simulink model "SDV_HIL"  (R2025a)
settings: Solver=VariableStepAuto  StartTime=0.0  StopTime=9999  FixedStep=0.001  RelTol=1e-3
undefined symbols (not defined in the file): Breakpoints_Fz, Cij, dspblkCoreblockFVToolHelper, eta, Fx_total_max, g, gcbh, Iz, lambda, lf, lr, mu, phi, R_eff, Tmax, xi
libraries: simulink_extras x30, slrealtimeiplib x17, slpidlib x16, simulink x10, SignalEditorBlockLib x6, dspstat3 x5, Solver_SF x3, sl3dlib x3
(part 5 of 5)

== matlab function SDV_HIL/Draft1/Steering Input1/Driver Logi G29/MATLAB Function ==
  data: btn input; state output
function state = fnc(btn)
%#codegen
% Start/Stop toggle dari 1 tombol joystick
% btn  : input tombol (0 atau 1, tipe double)
% state: output status (0=stop, 1=start)

persistent s last
if isempty(s)
    s = 0;      % status awal stop
    last = 0;   % tombol sebelumnya
end

% pastikan semua double
btn  = double(btn);
s    = double(s);
last = double(last);

% deteksi rising edge
if (btn == 1) && (last == 0)
    s = 1 - s;  % toggle
end

% simpan status tombol sebelumnya
last = btn;

% keluaran status
state = s;
end

== matlab function SDV_HIL/Draft1/UDP Receive ZCU -> PC1/MATLAB Function ==
  data: payload input; FL output; FR output; RL output; RR output; seqRecv output
function [FL, FR, RL, RR, seqRecv] = recvZCUFrame(payload)

% -------------------------------------------------------------------------
% recvZCUFrame
% Receive UDP frame from ZCU and decode per-wheel data
%
% Frame format (7 bytes):
% [1] Header = 0xCA
% [2] ID     = 1..4
% [3:4] Speed (int16)
% [5:6] Angle (int16)
% [7] Seq    (uint8)
% -------------------------------------------------------------------------

% =======================
% Persistent storage

persistent data
if isempty(data)
    % data(row,:) = [angle speed seq]
    data = zeros(4,3,'double');
end

% =======================
% Process incoming payload

data = processOne(payload, data);

% =======================
% Outputs

FL = data(1,1:2);
FR = data(2,1:2);
RL = data(3,1:2);
RR = data(4,1:2);

seqRecv = data(:,3);

% =======================
% Nested function

    function dataOut = processOne(payloadIn, dataIn)

        dataOut = dataIn;

        % Length check
        if numel(payloadIn) < 7
            return;
        end

        % Header check
        if payloadIn(1) ~= uint8(hex2dec('CB'))
            return;
        end

        % ID check
        id = payloadIn(2);
        if id < 1 || id > 4
            return;
        end

        % Decode
        speed = double(typecast(uint8(payloadIn(3:4)), 'int16'));
        angle = double(typecast(uint8(payloadIn(5:6)), 'int16'));
        seq   = double(payloadIn(7));

        dataOut(id,1) = speed;
        dataOut(id,2) = angle;
        dataOut(id,3) = seq;
    end
end

== matlab function SDV_HIL/Draft1/UDP Transmit PC -> VCU1/Subsystem/4 Wheel Steering system/Kinematik/4WS equation/MATLAB Function ==
  data: C1 input; of output; C2 input; R1 input; ir output; or output
function [of,ir,or] = fcn(C1, C2, R1)

of = 0;
ir = 0;
or = 0;
Hwt = 1.49/2;

of = rad2deg(atan(C1/(R1+Hwt)));
ir = rad2deg(atan(C2/(R1-Hwt)));
or = rad2deg(atan(C2/(R1+Hwt)));

== matlab function SDV_HIL/Draft1/UDP Transmit PC -> VCU1/Subsystem/4 Wheel Steering system/Kinematik/MATLAB Function ==
  data: if_deg input; fl output; of_deg input; ir_deg input; or_deg input; fr output; rl output; rr output
function [fl,fr,rl,rr] = fcn(if_deg,of_deg,ir_deg,or_deg)

if if_deg < 0
    fl = if_deg;
    fr = of_deg;
    rl = ir_deg;
    rr = or_deg;
elseif if_deg > 0
    fl = of_deg;
    fr = if_deg;
    rl = or_deg;
    rr = ir_deg;
else
    fl = 0;
    fr = 0;
    rl = 0;
    rr = 0;
end

== matlab function SDV_HIL/Draft1/UDP Transmit PC -> VCU1/Subsystem/4 Wheel Steering system/Kinematik/XO equation/MATLAB Function ==
  data: X0 output; Speed input; C2 output
function [X0,C2] = fcn(Speed)

CG = 1.55;
WheelBase = 3.1;

X0 = (Speed - CG) * (-1);
C2 = (Speed - WheelBase);

== matlab function SDV_HIL/Draft1/UDP Transmit PC -> VCU1/Subsystem/4 Wheel Steering system/Kinematik/YO equation/MATLAB Function ==
  data: Steer input; R1 output; Y0 output
function [R1,Y0] = fcn(Steer)

Hwb = 3.1/2;
Hwt = 1.49/2;
Y0 = 0;
R1 = 0;

k = tan(deg2rad(abs(Steer)));

if Steer == 0
    n = 0;
else
    n = k;
end

R1 = (Hwb/n)+Hwt;

if Steer > 0
    Y0 = R1;
elseif Steer < 0
    Y0 = R1*(-1);
else
    Y0 = 0;
end

== matlab function SDV_HIL/Draft1/UDP Transmit PC -> VCU1/Subsystem/MATLAB Function1 ==
  settings: updateMethod=DISCRETE
  data: TqMotor input; vxVehicle input; payload1 output; len1 output; vxWheel input; payload2 output; Throttle input; len2 output; angRef input; Mzd input; payload3 output; len3 output; payload4 output; len4 output
function [payload1, len1, payload2, len2, payload3, len3, payload4, len4] = ...
    packUDPFrame(TqMotor, vxVehicle, vxWheel, Throttle, angRef, Mzd)

% -------------------------------------------------------------------------
% packUDPFrame format 17 Byte:
% [0]  Header      uint8   = 0xCA
% [1]  ID          uint8   = 1..4 (FL, FR, RL, RR)
% [2]  TqWheel     int16
% [4]  vxVehicle   int16
% [6]  vxWheel     int16
% [8]  Throttle    int16
% [10] angRef      int16
% [12] Mzd         int32
% [16] seq         uint8
% 
% Only packing data into 4 UDP payloads (NO SENDING)
% Safe for Simulink Real-Time & Embedded Coder
% -------------------------------------------------------------------------

% =======================
% Constants

HEADER    = uint8(hex2dec('CA'));

% =======================
% Persistent sequence

persistent seq
if isempty(seq)
    seq = uint8(0);
end

% =======================
% Allocate outputs

payload1 = zeros(1,17,'uint8');
payload2 = zeros(1,17,'uint8');
payload3 = zeros(1,17,'uint8');
payload4 = zeros(1,17,'uint8');

% =======================
% Pack frames

payload1 = packOne(1, TqMotor(1), vxVehicle, vxWheel(1), Throttle, angRef(1), Mzd, seq);
payload2 = packOne(2, TqMotor(2), vxVehicle, vxWheel(2), Throttle, angRef(2), Mzd, seq);
payload3 = packOne(3, TqMotor(3), vxVehicle, vxWheel(3), Throttle, angRef(3), Mzd, seq);
payload4 = packOne(4, TqMotor(4), vxVehicle, vxWheel(4), Throttle, angRef(4), Mzd, seq);

% =======================
% Length outputs

len1 = uint8(numel(payload1));
len2 = uint8(numel(payload2));
len3 = uint8(numel(payload3));
len4 = uint8(numel(payload4));

% =======================
% Update sequence (0–255 loop)

seq = uint8(mod(double(seq) + 1, 256));

% =======================
% Nested packer

    function payload = packOne(id, tq, vxVeh, vxWh, thr, ang, mzd, sequence)

        payload = zeros(1,17,'uint8');

        payload(1) = HEADER;
        payload(2) = uint8(id);

        payload(3:4)   = typecast(int16(tq),  'uint8');
        payload(5:6)   = typecast(int16(vxVeh),  'uint8');
        payload(7:8)   = typecast(int16(vxWh),  'uint8');
        payload(9:10)  = typecast(int16(thr), 'uint8');
        payload(11:12) = typecast(int16(ang), 'uint8');
        payload(13:16) = typecast(int32(mzd), 'uint8');

        payload(17) = sequence;
    end
end

== matlab function SDV_HIL/Draft1/UDP Transmit PC -> VCU1/Subsystem/Torque Vectoring/Lower-Level Control/MATLAB Function1 ==
  data: lb output; ub output; Fx_total_ref input; Mx_total output; exitflag output; Mzd input; delta_in input; Fz input; Tshaft_max input; mu input; Fx_opt output; Fx_prev input
function [lb, ub, Mx_total, exitflag, Fx_opt] = torque_qp_mpc_function(Fx_total_ref, Mzd, delta_in, Fz, Tshaft_max, mu, Fx_prev)
%#codegen
% torque_qp_mpc_function - FINAL FIXED for Embedded Coder

%% 1. Persistent Memory & Varsize
persistent iA0_mem
if isempty(iA0_mem)
    iA0_mem = false(8, 1); 
end

% Definisi Variable Size untuk internal variables
coder.varsize('iA0_mem', [8 1], [1 0]); 
coder.varsize('iA_new',  [8 1], [1 0]);
coder.varsize('Fx_temp', [4 1], [1 0]); 

%% --- [FIXED STEP 1: Pre-allocate Output] ---
% Kita wajib mendefinisikan Fx_opt sebagai Fixed Size (4x1) di awal.
% Ini memberi tahu compiler: "Apapun yang terjadi, Fx_opt adalah 4x1".
Fx_opt = zeros(4,1); 

%% 2. Input Validation
assert(isreal(Mzd) && isscalar(Mzd));
assert(isreal(delta_in) && all(size(delta_in)==[2 1]));
assert(isreal(mu) && isscalar(mu));
assert(isreal(Fx_total_ref) && isscalar(Fx_total_ref));
assert(isreal(Fz) && all(size(Fz)==[4 1]));

%% 3. Vehicle Parameters
L = 4.595; lf = L/2; lr = L/2; df = 1.8; dr = 1.8;
Reff = 0.346; 

%% 4. Mx Coefficients
Mx_coeff = zeros(1,4);
Mx_coeff(1) = lf*sin(delta_in(1)) - (df/2)*cos(delta_in(1));
Mx_coeff(2) = lf*sin(delta_in(1)) + (df/2)*cos(delta_in(1));
Mx_coeff(3) = -lr*sin(delta_in(2)) - (dr/2)*cos(delta_in(2));
Mx_coeff(4) = -lr*sin(delta_in(2)) + (dr/2)*cos(delta_in(2));

%% 5. QP Cost (H, f)
n = 4;
Fz_safe = Fz.' + 1e-6; 
w = Mx_coeff ./ Fz_safe;                

H = 2 * diag(w.^2);
H = H + 1e-6 * eye(n); 
f = zeros(n, 1);

%% 6. Constraints
Aeq = [Mx_coeff; 1 1 1 1];
beq = [Mzd; Fx_total_ref];

Fx_max = min(Tshaft_max/Reff, mu .* Fz);
Fx_max = max(Fx_max, 0); 
lb = -Fx_max;
ub =  Fx_max;

A = [eye(n); -eye(n)];
b = [ub; -lb];

%% 7. Solver Options
persistent options
if isempty(options)
    options = mpcActiveSetOptions;    
    options.MaxIterations = int32(40);
    options.ConstraintTolerance = 1e-5;
    options.IntegrityChecks = false; 
    options.UseHessianAsInput = true; 
end

%% 8. Solve QP
[Fx_temp, exitflag, iA_new, ~] = mpcActiveSetSolver( ...
    H, f, A, b, Aeq, beq, iA0_mem, options);

%% --- [FIXED STEP 2: Explicit Index Assignment] ---
% Jangan gunakan "Fx_opt = Fx_temp" (itu membuat variable size menular).
% Gunakan indexing (1:4) untuk memaksa ukuran tetap.

if exitflag > 0 
    % Assignment elemen-ke-elemen memaksa ukuran tetap terjaga
    Fx_opt(1:4) = Fx_temp(1:4);
    
    iA0_mem = iA_new; 
else
    % Fallback
    Fx_opt(1:4) = Fx_prev(1:4);
end

%% 10. Output Calculation
% Mx_total juga akan aman karena Fx_opt sudah fixed
Mx_total = Mx_coeff * Fx_opt;

end

== matlab function SDV_HIL/HIL/UDP Transmit PC -> VCU/Subsystem/Torque Vectoring/Lower-Level Control/MATLAB Function1 ==
  data: lb output; ub output; Fx_total_ref input; Mx_total output; exitflag output; Mzd input; delta_in input; Fz input; Tshaft_max input; mu input; Fx_opt output; Fx_prev input
function [lb, ub, Mx_total, exitflag, Fx_opt] = torque_qp_mpc_function(Fx_total_ref, Mzd, delta_in, Fz, Tshaft_max, mu, Fx_prev)
%#codegen
% torque_qp_mpc_function - FINAL FIXED for Embedded Coder

%% 1. Persistent Memory & Varsize
persistent iA0_mem
if isempty(iA0_mem)
    iA0_mem = false(8, 1); 
end

% Definisi Variable Size untuk internal variables
coder.varsize('iA0_mem', [8 1], [1 0]); 
coder.varsize('iA_new',  [8 1], [1 0]);
coder.varsize('Fx_temp', [4 1], [1 0]); 

%% --- [FIXED STEP 1: Pre-allocate Output] ---
% Kita wajib mendefinisikan Fx_opt sebagai Fixed Size (4x1) di awal.
% Ini memberi tahu compiler: "Apapun yang terjadi, Fx_opt adalah 4x1".
Fx_opt = zeros(4,1); 

%% 2. Input Validation
assert(isreal(Mzd) && isscalar(Mzd));
assert(isreal(delta_in) && all(size(delta_in)==[2 1]));
assert(isreal(mu) && isscalar(mu));
assert(isreal(Fx_total_ref) && isscalar(Fx_total_ref));
assert(isreal(Fz) && all(size(Fz)==[4 1]));

%% 3. Vehicle Parameters
L = 4.595; lf = L/2; lr = L/2; df = 1.8; dr = 1.8;
Reff = 0.346; 

%% 4. Mx Coefficients
Mx_coeff = zeros(1,4);
Mx_coeff(1) = lf*sin(delta_in(1)) - (df/2)*cos(delta_in(1));
Mx_coeff(2) = lf*sin(delta_in(1)) + (df/2)*cos(delta_in(1));
Mx_coeff(3) = -lr*sin(delta_in(2)) - (dr/2)*cos(delta_in(2));
Mx_coeff(4) = -lr*sin(delta_in(2)) + (dr/2)*cos(delta_in(2));

%% 5. QP Cost (H, f)
n = 4;
Fz_safe = Fz.' + 1e-6; 
w = Mx_coeff ./ Fz_safe;                

H = 2 * diag(w.^2);
H = H + 1e-6 * eye(n); 
f = zeros(n, 1);

%% 6. Constraints
Aeq = [Mx_coeff; 1 1 1 1];
beq = [Mzd; Fx_total_ref];

Fx_max = min(Tshaft_max/Reff, mu .* Fz);
Fx_max = max(Fx_max, 0); 
lb = -Fx_max;
ub =  Fx_max;

A = [eye(n); -eye(n)];
b = [ub; -lb];

%% 7. Solver Options
persistent options
if isempty(options)
    options = mpcActiveSetOptions;    
    options.MaxIterations = int32(40);
    options.ConstraintTolerance = 1e-5;
    options.IntegrityChecks = false; 
    options.UseHessianAsInput = true; 
end

%% 8. Solve QP
[Fx_temp, exitflag, iA_new, ~] = mpcActiveSetSolver( ...
    H, f, A, b, Aeq, beq, iA0_mem, options);

%% --- [FIXED STEP 2: Explicit Index Assignment] ---
% Jangan gunakan "Fx_opt = Fx_temp" (itu membuat variable size menular).
% Gunakan indexing (1:4) untuk memaksa ukuran tetap.

if exitflag > 0 
    % Assignment elemen-ke-elemen memaksa ukuran tetap terjaga
    Fx_opt(1:4) = Fx_temp(1:4);
    
    iA0_mem = iA_new; 
else
    % Fallback
    Fx_opt(1:4) = Fx_prev(1:4);
end

%% 10. Output Calculation
% Mx_total juga akan aman karena Fx_opt sudah fixed
Mx_total = Mx_coeff * Fx_opt;

end

== matlab function SDV_HIL/HIL/UDP Transmit PC -> VCU/Subsystem/4 Wheel Steering system/Kinematik/4WS equation/MATLAB Function ==
  data: C1 input; of output; C2 input; R1 input; ir output; or output
function [of,ir,or] = fcn(C1, C2, R1)

of = 0;
ir = 0;
or = 0;
Hwt = 1.49/2;

of = rad2deg(atan(C1/(R1+Hwt)));
ir = rad2deg(atan(C2/(R1-Hwt)));
or = rad2deg(atan(C2/(R1+Hwt)));

== matlab function SDV_HIL/Draft1/UDP Transmit PC -> VCU1/Subsystem/Torque Vectoring/Reference Model/Draft/MATLAB Function1 ==
  data: AngWheel input; r output; Vx input
function r = fcn(AngWheel, Vx)

L       = 4.55;         % wheelbase
Vx = Vx / 3.6;          % km/h to m/s

Rr = L * cot(AngWheel);

r = Vx / Rr;

== matlab function SDV_HIL/Draft1/UDP Transmit PC -> VCU1/Subsystem/Torque Vectoring/Reference Model/Draft/MATLAB Function2 ==
  data: SteerAng input; Vx input; y output; Caf input; Car input
function y = fcn(SteerAng, Vx, Caf, Car)

% === EV Van Parameters ===
m_s     = 2380;         % sprung mass
m_us    = 392;          % unsprung mass
m       = m_s + m_us;   % vehicle mass
L       = 4.55;         % wheelbase
lf      = 2.184;         % wheel centers front to CoG
lr      = 2.366;         % wheel centers rear to CoG

Vx = Vx / 3.6;          % km/h to m/s

R = (L + ((m * Vx^2 * (lr*Car - lf*Caf)) / (Caf*Car*L))) / SteerAng;

e = -(lr/R) + ((lf*m*Vx^2) / (Car*L*R));

yawAng = e;
beta = -e;

y = [yawAng; beta];

== matlab function SDV_HIL/Draft1/UDP Transmit PC -> VCU1/Subsystem/Torque Vectoring/Reference Model/Reference Model ==
  data: delta_in input; Vx input; Caf input; y output; Car input
function y = fcn(delta_in, Vx, Caf, Car)

Vx_kmh = Vx; 
Vx_ms = Vx / 3.6;

L = 4.595; lf = L/2; lr = L/2; m = 2772;

if Vx_kmh > 3
    den = (L + ((m * Vx_ms^2 * (lr*Car - lf*Caf)) / (Caf * Car * L)));
    yawrate_des = (Vx_ms / den) * delta_in;
    beta_des    = ((lr - ((lf * m * Vx_ms^2) / (Car * L))) / den) * delta_in;
else
    yawrate_des = 0;
    beta_des    = 0;
end

y = [yawrate_des; beta_des];

== matlab function SDV_HIL/Draft1/UDP Transmit PC -> VCU1/Subsystem/Torque Vectoring/Speed Control/MATLAB Function ==
  data: Fx_total input; y output; Vx_des input; Vx input
function y = fcn(Fx_total, Vx_des, Vx)

if Vx_des > 1
    y = Fx_total;    
else
    y = 0;
end

== matlab function SDV_HIL/Draft1/VCU Com1/UDP Receive <- VCU1/MATLAB Function ==
  data: Steer output; Throttle output; Brake output; payload input; FL output; FR output; RL output; RR output; seqRef output; seqCalc output
function [Steer, Throttle, Brake, FL, FR, RL, RR, seqRef, seqCalc] = recvVCUFrame(payload)
% recvVCUFrame
% -------------------------------------------------------------------------
% Menerima data dari VCU melalui UDP.
%
% Mendukung 2 jenis frame:
% 1️⃣ Kalkulasi kendaraan (header=0xCA, ID=6, panjang=19 byte)
%    [Header, ID,
%     AngFL(2B), AngFR(2B), AngRL(2B), AngRR(2B),
%     SpdFL(2B), SpdFR(2B), SpdRL(2B), SpdRR(2B),
%     Seq(1B)]
%
% 2️⃣ Input driver (header=0xAA, ID=6, panjang=9 byte)
%    [Header, ID, Steer(2B), Throttle(2B), Brake(1B), Seq(1B)]
%
% Output:
%   FL, FR, RL, RR  : [angle speed] (1x2)
%   Steer, Throttle : scalar double
%   Brake           : scalar uint8/double
%   seqCalc, seqRef : sequence number masing-masing frame
% -------------------------------------------------------------------------

persistent data seqCalc_last seqRef_last steer_last throttle_last brake_last
if isempty(data)
    data = zeros(4,2,'double'); % [angle speed] tiap roda
    seqCalc_last = 0;
    seqRef_last = 0;
    steer_last = 0;
    throttle_last = 0;
    brake_last = 0;
end

% Default output (jika tidak ada data baru)
FL = data(1,:); FR = data(2,:);
RL = data(3,:); RR = data(4,:);
Steer = steer_last;
Throttle = throttle_last;
Brake = brake_last;
seqCalc = seqCalc_last;
seqRef = seqRef_last;

% Validasi payload
if isempty(payload) || numel(payload) < 3
    return;
end

header = payload(1);
id = payload(2);

switch header
    % =========================================================
    % === 1️⃣ FRAME CALCULATION DATA (Header 0xCA, len=19) ===
    % =========================================================
    case hex2dec('CA')
        if id == 6 && numel(payload) >= 19
            angFL = double(typecast(uint8(payload(3:4)), 'uint16'));
            angFR = double(typecast(uint8(payload(5:6)), 'uint16'));
            angRL = double(typecast(uint8(payload(7:8)), 'uint16'));
            angRR = double(typecast(uint8(payload(9:10)), 'uint16'));
            spdFL = double(typecast(uint8(payload(11:12)), 'uint16'));
            spdFR = double(typecast(uint8(payload(13:14)), 'uint16'));
            spdRL = double(typecast(uint8(payload(15:16)), 'uint16'));
            spdRR = double(typecast(uint8(payload(17:18)), 'uint16'));
            seq = double(payload(19));

            % Simpan hasilnya
            data(1,:) = [angFL, spdFL];
            data(2,:) = [angFR, spdFR];
            data(3,:) = [angRL, spdRL];
            data(4,:) = [angRR, spdRR];
            seqCalc_last = seq;
        end

    % =========================================================
    % === 2️⃣ FRAME DRIVER INPUT DATA (Header 0xAA, len=9) ===
    % =========================================================
    case hex2dec('AA')
        if id == 6 && numel(payload) >= 9
            steer    = double(typecast(uint8(payload(3:4)), 'uint16'));
            throttle = double(typecast(uint8(payload(5:6)), 'uint16'));
            brake    = double(payload(7));
            seq      = double(payload(8));

            steer_last = steer;
            throttle_last = throttle;
            brake_last = brake;
            seqRef_last = seq;
        end

    otherwise
        % Header tidak dikenali → abaikan
end

% Output terbaru
FL = data(1,:);
FR = data(2,:);
RL = data(3,:);
RR = data(4,:);
Steer = steer_last;
Throttle = throttle_last;
Brake = brake_last;
seqCalc = seqCalc_last;
seqRef = seqRef_last;

end

== matlab function SDV_HIL/Draft1/VCU Com1/UDP Send -> VCU1/MATLAB Function1 ==
  data: angWheel input; payload1 output; len1 output; spdWheel input; vxVehicle input; payload2 output; seqCalc input; len2 output
function [payload1, len1, payload2, len2] = sendUDPFrameSplit(angWheel, spdWheel, vxVehicle, seqCalc)
% sendUDPFrameSplit
% -------------------------------------------------------------------------
% Mengirim dua frame UDP:
%   1️⃣ Frame Feedback (Header=0xCA, ID=5)
%Frame Actual CarSim (Header=0xCE, ID=5)
%
% Input:
%   angWheel  : [1x4] sudut roda (FL, FR, RL, RR)
%   spdWheel  : [1x4] kecepatan roda (FL, FR, RL, RR)
%   vxVehicle : kecepatan longitudinal kendaraan
%   seqCalc   : sequence kalkulasi dari VCU
%
% Output:
%   payload1 : frame feedback (13 byte)
%   payload2 : frame actual carsim (19 byte)
%   len1, len2 : panjang payload masing-masing
% -------------------------------------------------------------------------

persistent seqFeedback
if isempty(seqFeedback)
    seqFeedback = uint8(0);
end

HEADER_FEEDBACK = uint8(hex2dec('CA'));
HEADER_ACTUAL   = uint8(hex2dec('CE'));
ID              = uint8(5);

%% === FRAME FEEDBACK ===
payload1 = zeros(1,13,'uint8');
payload1(1) = HEADER_FEEDBACK;
payload1(2) = ID;

% Angles (FL, FR, RL, RR)
payload1(3:4)   = typecast(uint16(angWheel(1)), 'uint8'); % FL
payload1(5:6)   = typecast(uint16(angWheel(2)), 'uint8'); % FR
payload1(7:8)   = typecast(uint16(angWheel(3)), 'uint8'); % RL
payload1(9:10)  = typecast(uint16(angWheel(4)), 'uint8'); % RR

% Vehicle longitudinal speed
payload1(11:12) = typecast(uint16(vxVehicle), 'uint8');

% Sequence feedback (auto increment)
payload1(13) = seqFeedback;

% Update feedback sequence (0→255→0)
seqFeedback = uint8(mod(double(seqFeedback) + 1, 256));

len1 = uint8(numel(payload1));

%% === FRAME ACTUAL CARSIM ===
payload2 = zeros(1,19,'uint8');
payload2(1) = HEADER_ACTUAL;
payload2(2) = ID;

% Angles
payload2(3:4)   = typecast(uint16(angWheel(1)), 'uint8'); % FL
payload2(5:6)   = typecast(uint16(angWheel(2)), 'uint8'); % FR
payload2(7:8)   = typecast(uint16(angWheel(3)), 'uint8'); % RL
payload2(9:10)  = typecast(uint16(angWheel(4)), 'uint8'); % RR

% Speeds
payload2(11:12) = typecast(uint16(spdWheel(1)), 'uint8'); % FL
payload2(13:14) = typecast(uint16(spdWheel(2)), 'uint8'); % FR
payload2(15:16) = typecast(uint16(spdWheel(3)), 'uint8'); % RL
payload2(17:18) = typecast(uint16(spdWheel(4)), 'uint8'); % RR

% Sequence dari input (seqCalc)
payload2(19) = uint8(seqCalc);

len2 = uint8(numel(payload2));

end

== matlab function SDV_HIL/HIL_VCU/UDP Receive Brake VCU -> PC/MATLAB Function ==
  data: payload input; Brake output; seqRecv output
function [Brake, seqRecv] = recvVCUBrake(payload)
% -------------------------------------------------------------------------
% recvVCUBrake
% Menerima frame khusus pengereman langsung dari VCU Linux
%
% Frame format (4 bytes):
% [1] Header = 0xCB
% [2] ID     = 0x06
% [3] Brake  (uint8)
% [4] Seq    (uint8)
% -------------------------------------------------------------------------

    % Simpan nilai terakhir jika paket yang datang salah/kosong
    persistent brake_val seq_val
    if isempty(brake_val)
        brake_val = 0;
        seq_val = 0;
    end
    
    % Validasi Ukuran (4 Byte), Header (0xCB), dan ID (0x06)
    if numel(payload) == 4 && payload(1) == uint8(hex2dec('CA')) && payload(2) == uint8(6)
        % Ekstrak payload
        brake_val = double(payload(3));
        seq_val   = double(payload(4));
    end
    
    % Output
    Brake   = brake_val;
    seqRecv = seq_val;
end

== matlab function SDV_HIL/HIL_VCU/UDP Receive ZCU -> PC/MATLAB Function ==
  data: payload input; FL output; FR output; RL output; RR output; seqRecv output
 function [FL, FR, RL, RR, seqRecv] = recvZCUFrame(payload)

% -------------------------------------------------------------------------
% recvZCUFrame
% Receive UDP frame from ZCU and decode per-wheel data
%
% Frame format (7 bytes):
% [1] Header = 0xBA
% [2] ID     = 1..4
% [3:4] Speed (int16)
% [5:6] Angle (int16)
% [7] Seq    (uint8)
% -------------------------------------------------------------------------

% =======================
% Persistent storage

persistent data
if isempty(data)
    % data(row,:) = [angle speed seq]
    data = zeros(4,3,'double');
end

% =======================
% Process incoming payload

data = processOne(payload, data);

% =======================

% Outputs

FL = data(1,1:2);
FR = data(2,1:2);
RL = data(3,1:2);
RR = data(4,1:2);

seqRecv = data(:,3);

% =======================

% Nested function

    function dataOut = processOne(payloadIn, dataIn)
        dataOut = dataIn;

        % Length check
        if numel(payloadIn) < 7
            return;
        end

        % Header check
        if payloadIn(1) ~= uint8(hex2dec('BA'))
            return;
        end

        % ID check
        id = payloadIn(2);
        if id < 1 || id > 4
            return;
        end

        % Decode
        speed = double(typecast(uint8(payloadIn(3:4)), 'int16'));
        angle = double(typecast(uint8(payloadIn(5:6)), 'int16'));
        seq   = double(payloadIn(7));

        dataOut(id,1) = speed;
        dataOut(id,2) = angle;
        dataOut(id,3) = seq;
    end
end

== matlab function SDV_HIL/HIL_VCU/UDP Transmit PC -> VCU/MATLAB Function1 ==
  settings: updateMethod=DISCRETE
  data: Vx input; Vy input; AngWheel input; r input; Fy input; Fz input; Vx_wheel input; payload output; len output
function [payload, len] = packVCUFrame(Vx, Vy, AngWheel, r, Fy, Fz, Vx_wheel)
% -------------------------------------------------------------------------
% Total Payload: 57 Bytes (Header + ID + Data + Seq)
% -------------------------------------------------------------------------

    HEADER = uint8(hex2dec('AC')); 
    ID     = uint8(5);             

    persistent seq
    if isempty(seq)
        seq = uint8(0);
    end

    payload = zeros(1, 57, 'uint8');

    % =========================================================
    % SCALING MATEMATIKA
    % =========================================================
    Vx_uint       = uint16(Vx * 100);
    Vy_uint       = uint16((Vy + 10.0) * 100);
    
    Ang_uint      = uint16((AngWheel + 0.7) * 1000); % Array 1x4
    r_uint        = uint16((r + 0.7) * 1000);
    
    Fy_uint       = uint32((Fy + 9000.0) * 10);      % Array 1x4
    Fz_uint       = uint32(Fz * 10);                 % Array 1x4
    
    Vx_wheel_uint = uint16(Vx_wheel * 100);          % Array 1x4

    % =========================================================
    % PACKING BYTE
    % =========================================================
    payload(1) = HEADER;
    payload(2) = ID;

    payload(3:4)   = typecast(Vx_uint, 'uint8');
    payload(5:6)   = typecast(Vy_uint, 'uint8');

    payload(7:8)   = typecast(Ang_uint(1), 'uint8');
    payload(9:10)  = typecast(Ang_uint(2), 'uint8');
    payload(11:12) = typecast(Ang_uint(3), 'uint8');
    payload(13:14) = typecast(Ang_uint(4), 'uint8');

    payload(15:16) = typecast(r_uint, 'uint8');

    payload(17:20) = typecast(Fy_uint(1), 'uint8');
    payload(21:24) = typecast(Fy_uint(2), 'uint8');
    payload(25:28) = typecast(Fy_uint(3), 'uint8');
    payload(29:32) = typecast(Fy_uint(4), 'uint8');

    payload(33:36) = typecast(Fz_uint(1), 'uint8');
    payload(37:40) = typecast(Fz_uint(2), 'uint8');
    payload(41:44) = typecast(Fz_uint(3), 'uint8');
    payload(45:48) = typecast(Fz_uint(4), 'uint8');

    payload(49:50) = typecast(Vx_wheel_uint(1), 'uint8');
    payload(51:52) = typecast(Vx_wheel_uint(2), 'uint8');
    payload(53:54) = typecast(Vx_wheel_uint(3), 'uint8');
    payload(55:56) = typecast(Vx_wheel_uint(4), 'uint8');

    payload(57) = seq;

    % =========================================================
    % OUTPUT & SEQUENCE UPDATE
    % =========================================================
    len = uint8(57);
    seq = uint8(mod(double(seq) + 1, 256));
end

== matlab function SDV_HIL/HIL/UDP Transmit PC -> VCU/Subsystem/4 Wheel Steering system/Kinematik/MATLAB Function ==
  data: if_deg input; fl output; of_deg input; ir_deg input; or_deg input; fr output; rl output; rr output
function [fl,fr,rl,rr] = fcn(if_deg,of_deg,ir_deg,or_deg)

if if_deg < 0
    fl = if_deg;
    fr = of_deg;
    rl = ir_deg;
    rr = or_deg;
elseif if_deg > 0
    fl = of_deg;
    fr = if_deg;
    rl = or_deg;
    rr = ir_deg;
else
    fl = 0;
    fr = 0;
    rl = 0;
    rr = 0;
end

== matlab function SDV_HIL/HIL/UDP Transmit PC -> VCU/Subsystem/4 Wheel Steering system/Kinematik/XO equation/MATLAB Function ==
  data: X0 output; Speed input; C2 output
function [X0,C2] = fcn(Speed)

CG = 1.55;
WheelBase = 3.1;

X0 = (Speed - CG) * (-1);
C2 = (Speed - WheelBase);

== matlab function SDV_HIL/HIL/UDP Transmit PC -> VCU/Subsystem/Torque Vectoring/Reference Model/Draft/MATLAB Function1 ==
  data: AngWheel input; r output; Vx input
function r = fcn(AngWheel, Vx)

L       = 4.55;         % wheelbase
Vx = Vx / 3.6;          % km/h to m/s

Rr = L * cot(AngWheel);

r = Vx / Rr;

== matlab function SDV_HIL/HIL/UDP Transmit PC -> VCU/Subsystem/Torque Vectoring/Reference Model/Draft/MATLAB Function2 ==
  data: SteerAng input; Vx input; y output; Caf input; Car input
function y = fcn(SteerAng, Vx, Caf, Car)

% === EV Van Parameters ===
m_s     = 2380;         % sprung mass
m_us    = 392;          % unsprung mass
m       = m_s + m_us;   % vehicle mass
L       = 4.55;         % wheelbase
lf      = 2.184;         % wheel centers front to CoG
lr      = 2.366;         % wheel centers rear to CoG

Vx = Vx / 3.6;          % km/h to m/s

R = (L + ((m * Vx^2 * (lr*Car - lf*Caf)) / (Caf*Car*L))) / SteerAng;

e = -(lr/R) + ((lf*m*Vx^2) / (Car*L*R));

yawAng = e;
beta = -e;

y = [yawAng; beta];

== matlab function SDV_HIL/HIL/UDP Transmit PC -> VCU/Subsystem/Torque Vectoring/Reference Model/Reference Model ==
  data: delta_in input; Vx input; Caf input; y output; Car input
function y = fcn(delta_in, Vx, Caf, Car)

Vx_kmh = Vx; 
Vx_ms = Vx / 3.6;

L = 4.595; lf = L/2; lr = L/2; m = 2772;

if Vx_kmh > 3
    den = (L + ((m * Vx_ms^2 * (lr*Car - lf*Caf)) / (Caf * Car * L)));
    yawrate_des = (Vx_ms / den) * delta_in;
    beta_des    = ((lr - ((lf * m * Vx_ms^2) / (Car * L))) / den) * delta_in;
else
    yawrate_des = 0;
    beta_des    = 0;
end

y = [yawrate_des; beta_des];

== matlab function SDV_HIL/HIL/UDP Transmit PC -> VCU/Subsystem/MATLAB Function1 ==
  settings: updateMethod=DISCRETE
  data: TqMotor input; vxVehicle input; payload1 output; len1 output; vxWheel input; payload2 output; Throttle input; len2 output; angRef input; Mzd input; payload3 output; len3 output; payload4 output; len4 output
function [payload1, len1, payload2, len2, payload3, len3, payload4, len4] = ...
    packUDPFrame(TqMotor, vxVehicle, vxWheel, Throttle, angRef, Mzd)

% -------------------------------------------------------------------------
% packUDPFrame format 17 Byte:
% [0]  Header      uint8   = 0xCA
% [1]  ID          uint8   = 1..4 (FL, FR, RL, RR)
% [2]  TqWheel     int16
% [4]  vxVehicle   int16
% [6]  vxWheel     int16
% [8]  Throttle    int16
% [10] angRef      int16
% [12] Mzd         int32
% [16] seq         uint8
% 
% Only packing data into 4 UDP payloads (NO SENDING)
% Safe for Simulink Real-Time & Embedded Coder
% -------------------------------------------------------------------------

% =======================
% Constants

HEADER    = uint8(hex2dec('CA'));

% =======================
% Persistent sequence

persistent seq
if isempty(seq)
    seq = uint8(0);
end

% =======================
% Allocate outputs

payload1 = zeros(1,17,'uint8');
payload2 = zeros(1,17,'uint8');
payload3 = zeros(1,17,'uint8');
payload4 = zeros(1,17,'uint8');

% =======================
% Pack frames

payload1 = packOne(1, TqMotor(1), vxVehicle, vxWheel(1), Throttle, angRef(1), Mzd, seq);
payload2 = packOne(2, TqMotor(2), vxVehicle, vxWheel(2), Throttle, angRef(2), Mzd, seq);
payload3 = packOne(3, TqMotor(3), vxVehicle, vxWheel(3), Throttle, angRef(3), Mzd, seq);
payload4 = packOne(4, TqMotor(4), vxVehicle, vxWheel(4), Throttle, angRef(4), Mzd, seq);

% =======================
% Length outputs

len1 = uint8(numel(payload1));
len2 = uint8(numel(payload2));
len3 = uint8(numel(payload3));
len4 = uint8(numel(payload4));

% =======================
% Update sequence (0–255 loop)

seq = uint8(mod(double(seq) + 1, 256));

% =======================
% Nested packer

    function payload = packOne(id, tq, vxVeh, vxWh, thr, ang, mzd, sequence)

        payload = zeros(1,17,'uint8');

        payload(1) = HEADER;
        payload(2) = uint8(id);

        payload(3:4)   = typecast(int16(tq),  'uint8');
        payload(5:6)   = typecast(int16(vxVeh),  'uint8');
        payload(7:8)   = typecast(int16(vxWh),  'uint8');
        payload(9:10)  = typecast(int16(thr), 'uint8');
        payload(11:12) = typecast(int16(ang), 'uint8');
        payload(13:16) = typecast(int32(mzd), 'uint8');

        payload(17) = sequence;
    end
end
